simulink model "TireMagicFormula_R2025b"  (R2025b)
settings: Solver=FixedStepDiscrete  StartTime=0.0  StopTime=5  FixedStep=0.001  RelTol=1e-3
settings Model: Creator=12482  LastModifiedBy=12482

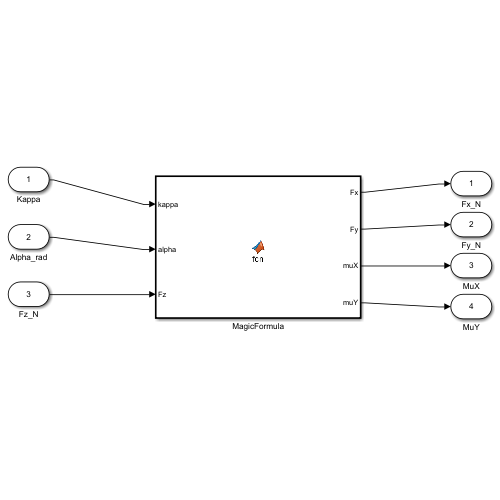
[thumbnail: Simulink's stored preview of the top-level diagram]
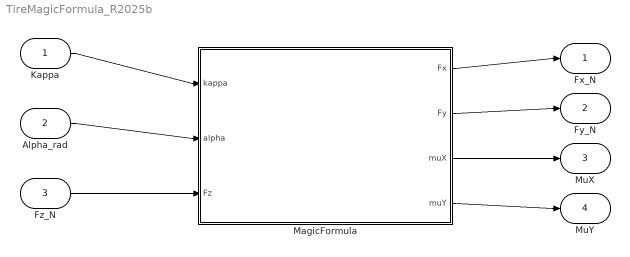
== system TireMagicFormula_R2025b ==
  Kappa : Inport
  Alpha_rad : Inport  Port=2
  Fz_N : Inport  Port=3
  MagicFormula : MATLAB Function  TreatAsAtomicUnit=on
  Fx_N : Outport
  Fy_N : Outport  Port=2
  MuX : Outport  Port=3
  MuY : Outport  Port=4
  wires:
  Kappa/1 -> MagicFormula/1(kappa)
  Alpha_rad/1 -> MagicFormula/2(alpha)
  Fz_N/1 -> MagicFormula/3(Fz)
  MagicFormula/1(Fx) -> Fx_N/1
  MagicFormula/2(Fy) -> Fy_N/1
  MagicFormula/3(muX) -> MuX/1
  MagicFormula/4(muY) -> MuY/1

== matlab function TireMagicFormula_R2025b/MagicFormula ==
  data: kappa input; Fx output; alpha input; Fz input; Fy output; muX output; muY output
function [Fx,Fy,muX,muY] = fcn(kappa,alpha,Fz)
%#codegen
Fz = max(Fz,0);
Fz0 = 4000.0;
Bx = 10.0; Cx = 1.65; Ex = 0.97; muX0 = 1.05;
By = 7.0;  Cy = 1.30; Ey = -1.60; muY0 = 1.00;
muLoadX = -0.08; muLoadY = -0.10;
lr = max(Fz/Fz0,1e-6);
muX = muX0*lr^muLoadX;
muY = muY0*lr^muLoadY;
Dx = muX*Fz;
Dy = muY*Fz;

zx = kappa;
Bxz = Bx*zx;
Fx0 = Dx*sin(Cx*atan(Bxz-Ex*(Bxz-atan(Bxz))));

zy = alpha;
Byz = By*zy;
Fy0 = Dy*sin(Cy*atan(Byz-Ey*(Byz-atan(Byz))));

nx = Fx0/max(abs(Dx),1e-9);
ny = Fy0/max(abs(Dy),1e-9);
normF = sqrt(nx*nx + ny*ny);
scale = 1.0;
if normF > 1.0
    scale = 1.0/normF;
end
Fx = Fx0*scale;
Fy = Fy0*scale;
end
